simulink model "QUESTION3_22"  (R2021a)
settings: Solver=VariableStepAuto  StartTime=0.0  StopTime=10.0  RelTol=1e-3
settings Model: Creator=user  LastModifiedBy=user

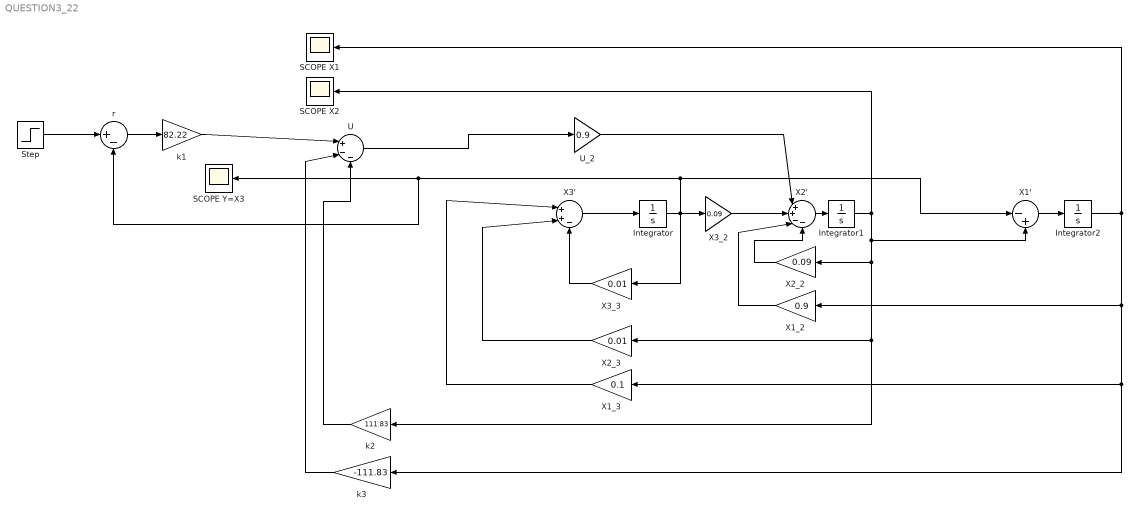
== system QUESTION3_22 ==
  Integrator : Integrator
  Integrator1 : Integrator
  Integrator2 : Integrator
  SCOPE X1 : Scope
  SCOPE X2 : Scope
  SCOPE Y=X3 : Scope
  Step : Step  SampleTime=0
  U : Sum  Inputs=|+--
  U_2 : Gain  Gain=0.9
  X1' : Sum  Inputs=|-+
  X1_2 : Gain  Gain=0.9
  X1_3 : Gain  Gain=0.1
  X2' : Sum  Inputs=|++--
  X2_2 : Gain  Gain=0.09
  X2_3 : Gain  Gain=0.01
  X3' : Sum  Inputs=|++-
  X3_2 : Gain  Gain=0.09
  X3_3 : Gain  Gain=0.01
  k1 : Gain  Gain=82.22
  k2 : Gain  Gain=111.83
  k3 : Gain  Gain=-111.83
  r : Sum  Inputs=|+-
  wires:
  X1_3/1 -> X3'/1
  X3'/1 -> Integrator/1
  Integrator1/1 -> X2_3/1, k2/1, X2_2/1, X1'/2, SCOPE X2/1
  X1'/1 -> Integrator2/1
  X2'/1 -> Integrator1/1
  Integrator/1 -> X3_3/1, X1'/1, r/2, SCOPE Y=X3/1, X3_2/1
  X2_3/1 -> X3'/2
  X3_3/1 -> X3'/3
  Integrator2/1 -> SCOPE X1/1, X1_2/1, k3/1, X1_3/1
  X3_2/1 -> X2'/2
  U_2/1 -> X2'/1
  X2_2/1 -> X2'/4
  X1_2/1 -> X2'/3
  Step/1 -> r/1
  r/1 -> k1/1
  k1/1 -> U/1
  U/1 -> U_2/1
  k3/1 -> U/2
  k2/1 -> U/3
